simulink model "untitled"  (R2020b)
settings: Solver=VariableStepAuto  StartTime=0.0  StopTime=10.0  RelTol=1e-3
values from neighbouring files (symbols this model uses):
  A = [0 1 0 0 0;0 0 0 0 0;0 0 0 0 0;1 0 0 0 0;0 0 1 0 0]    [init_heli_3_10.m]
  B = [0 0; 0 K_1; K_2 0;0 0;0 0]    [init_heli_3_10.m]
  F = [K(1,1), K(1,3); K(2,1), K(2,3)]    [init_heli_3_10.m]
  G = [0 0;0 0;0 0;-1 0;0 -1]    [init_heli_3_10.m]
  K = lqr(A, B, Q, R)    [init_heli_3_10.m]
settings Model: Creator=erlin  LastModifiedBy=erlin

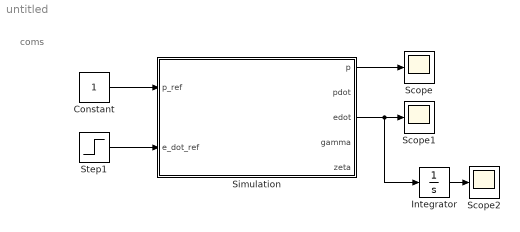
== system untitled ==
  note: coms
  Constant : Constant
  Integrator : Integrator
  Scope : Scope
  Scope1 : Scope
  Scope2 : Scope
  Simulation : Subsystem
  Step1 : Step  Time=2  Before=1  After=0  SampleTime=0
  wires:
  Step1/1 -> Simulation/2(e_dot_ref)
  Constant/1 -> Simulation/1(p_ref)
  Simulation/1(p) -> Scope/1
  Simulation/3(edot) -> Integrator/1, Scope1/1
  Integrator/1 -> Scope2/1

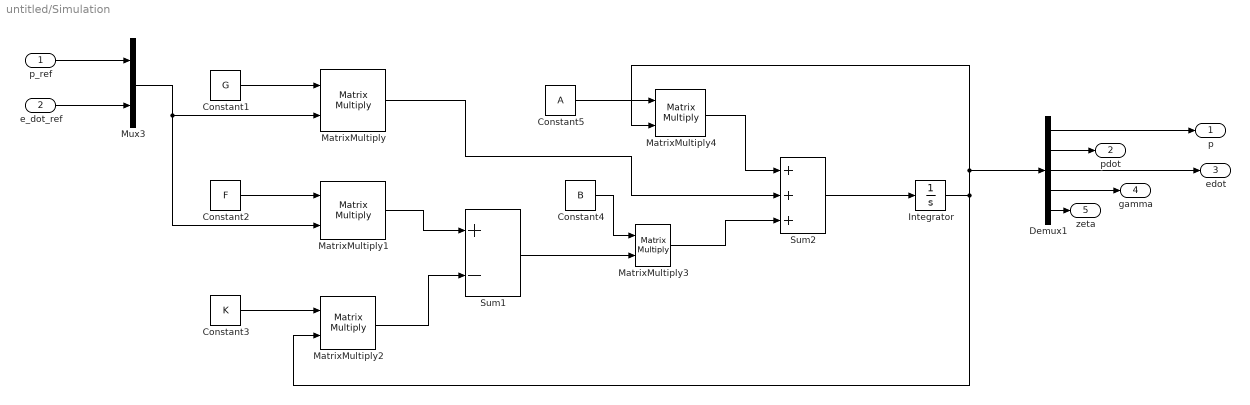
== system untitled/Simulation ==
  p_ref : Inport
  e_dot_ref : Inport  Port=2
  Constant1 : Constant  Value=G
  Constant2 : Constant  Value=F
  Constant3 : Constant  Value=K
  Constant4 : Constant  Value=B
  Constant5 : Constant  Value=A
  Demux1 : Demux  Outputs=5
  Integrator : Integrator
  MatrixMultiply{,1..4} (5 alike) : Product  Multiplication=Matrix(*)
  Mux3 : Mux  Inputs=2
  Sum1 : Sum  Inputs=+-
  Sum2 : Sum  Inputs=+++
  p : Outport
  pdot : Outport  Port=2
  edot : Outport  Port=3
  gamma : Outport  Port=4
  zeta : Outport  Port=5
  wires:
  Constant2/1 -> MatrixMultiply1/1
  Constant5/1 -> MatrixMultiply4/1
  Sum2/1 -> Integrator/1
  Constant4/1 -> MatrixMultiply3/1
  Integrator/1 -> MatrixMultiply4/2, Demux1/1, MatrixMultiply2/2
  Demux1/5 -> zeta/1
  Constant1/1 -> MatrixMultiply/1
  MatrixMultiply2/1 -> Sum1/2
  MatrixMultiply/1 -> Sum2/2
  Mux3/1 -> MatrixMultiply1/2, MatrixMultiply/2
  MatrixMultiply1/1 -> Sum1/1
  MatrixMultiply4/1 -> Sum2/1
  Constant3/1 -> MatrixMultiply2/1
  Sum1/1 -> MatrixMultiply3/2
  Demux1/3 -> edot/1
  MatrixMultiply3/1 -> Sum2/3
  Demux1/1 -> p/1
  e_dot_ref/1 -> Mux3/2
  p_ref/1 -> Mux3/1
  Demux1/2 -> pdot/1
  Demux1/4 -> gamma/1
